simulink library "VelocityController_v3_CL"  (R2020a)
settings: Solver=VariableStepAuto  StartTime=0.0  StopTime=10.0  RelTol=1e-3
libraries: Thesis_Sublibraries x5, MPC_51_v3_GP_CL x1
settings Model: Creator=John Jr  LastModifiedBy=John Jr

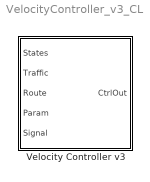
== system VelocityController_v3_CL ==
  Velocity Controller v3 : Subsystem  TreatAsAtomicUnit=on
      mask Display:
      | patch([0 1 1 0], [0 0 1 1],[1 .8 1])
      | 
      | port_label('input',1,'\fontname{Cambria Math}States','texmode','on')
      | port_label('input',2,'\fontname{Cambria Math}Traffic','texmode','on')
      | port_label('input',3,'\fontname{Cambria Math}Route','texmode','on')
      | port_label('input',4,'\fontname{Cambria Math}Param','texmode','on')
      | port_label('input',5,'\fontname{Cambria Math}Signal','texmode','on')
      | 
      | port_label('output',1,'\fontname{Cambria Math}CtrlOut','texmode','on')

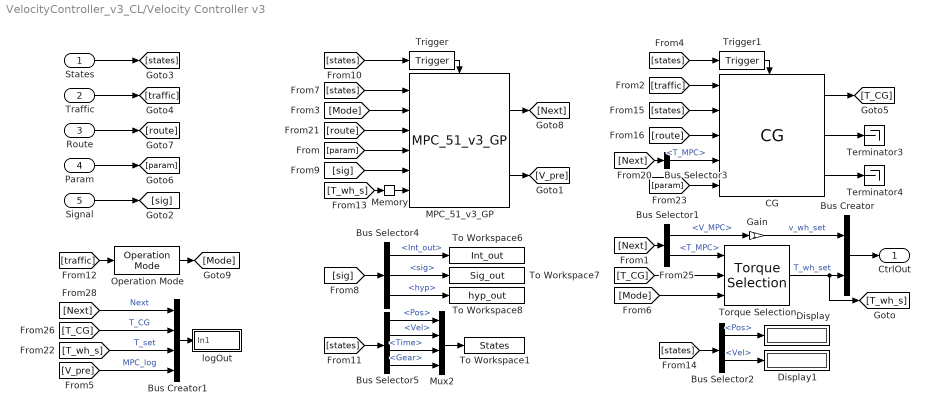
== system VelocityController_v3_CL/Velocity Controller v3 ==
  States : Inport
  Traffic : Inport  Port=2
  Route : Inport  Port=3
  Param : Inport  Port=4
  Signal : Inport  Port=5
  Bus Creator : BusCreator  Inputs=2
  Bus Creator1 : BusCreator  Inputs=4
  Bus Selector1 : BusSelector  OutputSignals=V_MPC,T_MPC
  Bus Selector2 : BusSelector  OutputSignals=Pos,Vel
  Bus Selector3 : BusSelector  OutputSignals=T_MPC
  Bus Selector4 : BusSelector  OutputSignals=Int_out,sig,hyp
  Bus Selector5 : BusSelector  OutputSignals=Pos,Vel,Time,Gear
  CG : Thesis_Sublibraries/CG  SystemSampleTime=-1  Latency=0  AutoFrameSizeCalculation=off
  Display : Display
  Display1 : Display
  Gain : Gain
  MPC_51_v3_GP : MPC_51_v3_GP_CL/MPC_51_v3_GP  SystemSampleTime=-1  Latency=0  AutoFrameSizeCalculation=off
  Memory : Memory  InitialCondition=11
  Mux2 : Mux
  Operation Mode : Thesis_Sublibraries/Operation Mode  ds_max=200
  Terminator3 : Terminator
  Terminator4 : Terminator
  To Workspace1 : ToWorkspace  VariableName=States  SampleTime=-1
  To Workspace6 : ToWorkspace  VariableName=Int_out  SampleTime=-1
  To Workspace7 : ToWorkspace  VariableName=Sig_out  SampleTime=-1
  To Workspace8 : ToWorkspace  VariableName=hyp_out  SampleTime=-1
  Torque Selection : Thesis_Sublibraries/Torque Selection  SystemSampleTime=-1  Latency=0  AutoFrameSizeCalculation=off
  Trigger : Thesis_Sublibraries/Trigger  f=1
  Trigger1 : Thesis_Sublibraries/Trigger  f=2.5
  logOut : Subsystem
      mask Display:
      | patch([0 1 1 0], [0 0 1 1],[.8 1 .8])
      | 
      | port_label('input',1,'Log Out')
  CtrlOut : Outport  VectorParamsAs1DForOutWhenUnconnected=off
  wires:
  Traffic/1 -> [traffic]
  Route/1 -> [route]
  States/1 -> [states]
  [states] -> Trigger/1
  Trigger/1 -> MPC_51_v3_GP/Trigger
  [route] -> MPC_51_v3_GP/3
  [param] -> MPC_51_v3_GP/4
  [Mode] -> MPC_51_v3_GP/2
  [states] -> MPC_51_v3_GP/1
  Param/1 -> [param]
  MPC_51_v3_GP/1 -> [Next]
  Gain/1 -> Bus Creator/1  "v_wh_set"
  Bus Selector1/1 -> Gain/1  "<V_MPC>"
  Bus Selector1/2 -> Torque Selection/1  "<T_MPC>"
  [Mode] -> Torque Selection/3
  [Next] -> Bus Selector1/1
  Torque Selection/1 -> [T_wh_s], Bus Creator/2  "T_wh_set"
  [T_CG] -> Torque Selection/2
  Bus Creator/1 -> CtrlOut/1
  CG/3 -> Terminator4/1
  [Next] -> Bus Selector3/1
  [param] -> CG/5
  CG/1 -> [T_CG]
  Bus Selector3/1 -> CG/4  "<T_MPC>"
  [route] -> CG/3
  Trigger1/1 -> CG/Trigger
  [states] -> Trigger1/1
  CG/2 -> Terminator3/1
  [states] -> CG/2
  [traffic] -> CG/1
  [V_pre] -> Bus Creator1/4  "MPC_log"
  [T_CG] -> Bus Creator1/2  "T_CG"
  [T_wh_s] -> Bus Creator1/3  "T_set"
  [Next] -> Bus Creator1/1  "Next"
  Bus Creator1/1 -> logOut/1(In1)
  Signal/1 -> [sig]
  MPC_51_v3_GP/2 -> [V_pre]
  [sig] -> MPC_51_v3_GP/5
  Memory/1 -> MPC_51_v3_GP/6
  [T_wh_s] -> Memory/1
  Bus Selector2/1 -> Display/1  "<Pos>"
  [states] -> Bus Selector2/1
  Bus Selector2/2 -> Display1/1  "<Vel>"
  [sig] -> Bus Selector4/1
  Bus Selector4/1 -> To Workspace6/1  "<Int_out>"
  Bus Selector4/3 -> To Workspace8/1  "<hyp>"
  Bus Selector4/2 -> To Workspace7/1  "<sig>"
  Bus Selector5/4 -> Mux2/4  "<Gear>"
  Bus Selector5/1 -> Mux2/1  "<Pos>"
  Mux2/1 -> To Workspace1/1
  Bus Selector5/2 -> Mux2/2  "<Vel>"
  Bus Selector5/3 -> Mux2/3  "<Time>"
  [states] -> Bus Selector5/1
  [traffic] -> Operation Mode/1
  Operation Mode/1 -> [Mode]

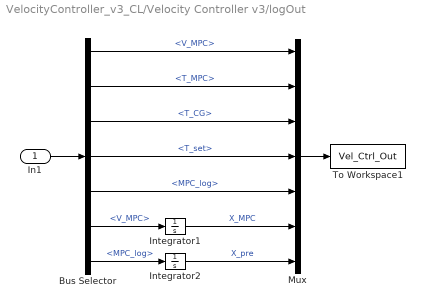
== system VelocityController_v3_CL/Velocity Controller v3/logOut ==
  In1 : Inport
  Bus Selector : BusSelector  OutputSignals=Next.V_MPC,Next.T_MPC,T_CG,T_set,MPC_log,Next.V_MPC,MPC_log
  Integrator1 : Integrator
  Integrator2 : Integrator
  Mux : Mux  Inputs=7
  To Workspace1 : ToWorkspace  VariableName=Vel_Ctrl_Out  SaveFormat=Structure With Time  SampleTime=-1
  wires:
  Bus Selector/4 -> Mux/4  "<T_set>"
  Bus Selector/3 -> Mux/3  "<T_CG>"
  Bus Selector/2 -> Mux/2  "<T_MPC>"
  Bus Selector/1 -> Mux/1  "<V_MPC>"
  Mux/1 -> To Workspace1/1
  In1/1 -> Bus Selector/1
  Bus Selector/5 -> Mux/5  "<MPC_log>"
  Bus Selector/6 -> Integrator1/1  "<V_MPC>"
  Bus Selector/7 -> Integrator2/1  "<MPC_log>"
  Integrator1/1 -> Mux/6  "X_MPC"
  Integrator2/1 -> Mux/7  "X_pre"
